simulink model "pro"  (R2012b)
settings: Solver=ode45  StartTime=0.0  StopTime=3  FixedStep=0.001  RelTol=1e-1  AbsTol=1e-2
undefined symbols (not defined in the file or in its folder): v_max
libraries: simulink x2
settings Model: Creator=Milos  LastModifiedBy=Caka
settings SolverCC: MaxConsecutiveMinStep=5

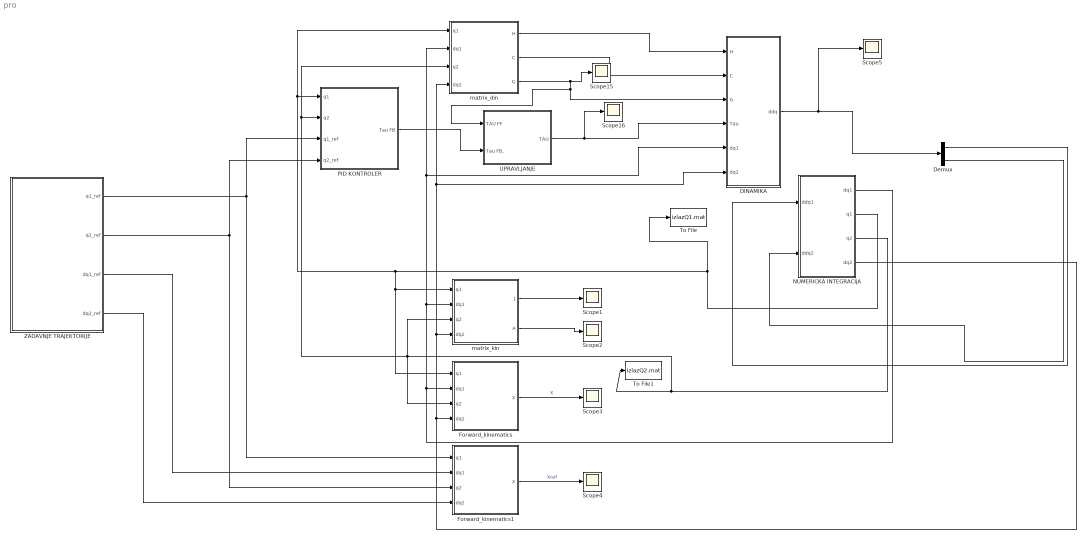
== system pro ==
  DINAMIKA : Subsystem
  Demux : Demux  Outputs=2
  Forward_kinematics : Subsystem
  Forward_kinematics1 : Subsystem
  NUMERICKA INTEGRACIjA : Subsystem
  PID KONTROLER : Subsystem
  Scope{1..5,15..16} (7 alike) : Scope
      Scope1 settings: TimeRange=5  YMin=0  YMax=70  SaveName=ScopeData4
      Scope15 settings: TimeRange=5  YMin=0  YMax=70  SaveName=ScopeData19
      Scope16 settings: TimeRange=5  YMin=0  YMax=70  SaveName=ScopeData20
      Scope2 settings: TimeRange=5  YMin=0  YMax=70  SaveName=ScopeData5
      Scope3 settings: TimeRange=5  YMin=0  YMax=70  SaveName=ScopeData6
      Scope4 settings: TimeRange=5  YMin=0  YMax=70  SaveName=ScopeData7
      Scope5 settings: TimeRange=5  YMin=0  YMax=70  SaveName=ScopeData9
  To File : ToFile  Filename=izlazQ1.mat  MatrixName=q1  SampleTime=0.01
  To File1 : ToFile  Filename=izlazQ2.mat  MatrixName=q2  SampleTime=0.01
  UPRAVLJANJE : Subsystem
  ZADAVNJE TRAJEKTORIJE : Subsystem
  matrix_din : Subsystem
  matrix_kin : Subsystem
  wires:
  matrix_din/3(G) -> Scope15/1, DINAMIKA/3(G), UPRAVLJANJE/1(TAU FF)
  matrix_kin/1(J) -> Scope1/1
  matrix_kin/2(A) -> Scope2/1
  Forward_kinematics/1(X) -> Scope3/1  "X"
  Forward_kinematics1/1(X) -> Scope4/1  "Xref"
  ZADAVNJE TRAJEKTORIJE/1(q1_ref) -> PID KONTROLER/3(q1_ref), Forward_kinematics1/1(q1)
  ZADAVNJE TRAJEKTORIJE/4(dq2_ref) -> Forward_kinematics1/4(dq2)
  matrix_din/1(H) -> DINAMIKA/1(H)
  matrix_din/2(C) -> DINAMIKA/2(C)
  UPRAVLJANJE/1(TAU) -> Scope16/1, DINAMIKA/4(Tau)
  PID KONTROLER/1("Tau FB ") -> UPRAVLJANJE/2(Tau FB,)
  ZADAVNJE TRAJEKTORIJE/2(q2_ref) -> PID KONTROLER/4(q2_ref), Forward_kinematics1/3(q2)
  ZADAVNJE TRAJEKTORIJE/3(dq1_ref) -> Forward_kinematics1/2(dq1)
  NUMERICKA INTEGRACIjA/4(dq2) -> Forward_kinematics/4(dq2), DINAMIKA/6(dq2), matrix_din/4(dq2), matrix_kin/4(dq2)
  NUMERICKA INTEGRACIjA/2(q1) -> Forward_kinematics/1(q1), matrix_kin/1(q1), matrix_din/1(q1), PID KONTROLER/1(q1), To File/1
  NUMERICKA INTEGRACIjA/3(q2) -> To File1/1, PID KONTROLER/2(q2), matrix_din/3(q2), matrix_kin/3(q2), Forward_kinematics/3(q2)
  Demux/1 -> NUMERICKA INTEGRACIjA/1(ddq1)
  Demux/2 -> NUMERICKA INTEGRACIjA/2(ddq2)
  NUMERICKA INTEGRACIjA/1(dq1) -> DINAMIKA/5(dq1), matrix_din/2(dq1), matrix_kin/2(dq1), Forward_kinematics/2(dq1)
  DINAMIKA/1(ddq) -> Scope5/1, Demux/1

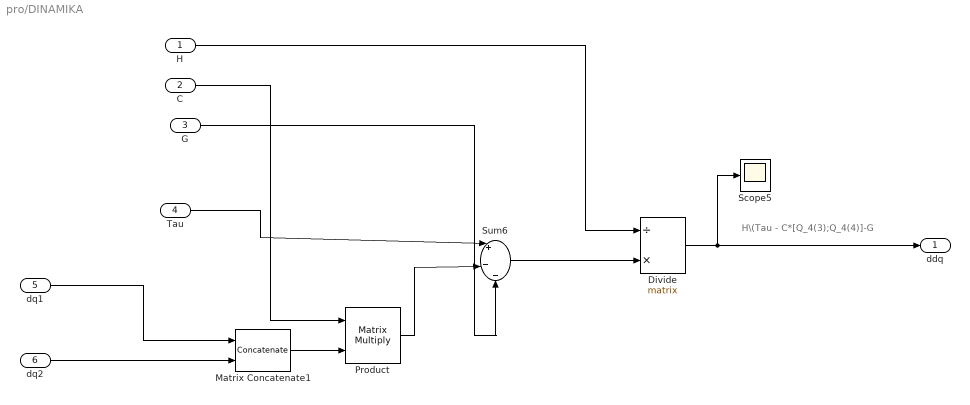
== system pro/DINAMIKA ==
  note: H\(Tau - C*[Q_4(3);Q_4(4)]-G
  H : Inport
  C : Inport  Port=2
  G : Inport  Port=3
  Tau : Inport  Port=4
  dq1 : Inport  Port=5
  dq2 : Inport  Port=6
  Divide : Product  Inputs=/*  Multiplication=Matrix(*)
  Matrix Concatenate1 : Concatenate  Mode=Multidimensional array
  Product : Product  Multiplication=Matrix(*)  RndMeth=Zero
  Scope5 : Scope
      settings: TimeRange=5  YMin=0  YMax=70  SaveName=ScopeData8
  Sum6 : Sum  Inputs=|+|-|-
  ddq : Outport
  wires:
  Product/1 -> Sum6/2
  H/1 -> Divide/1
  Matrix Concatenate1/1 -> Product/2
  Sum6/1 -> Divide/2
  C/1 -> Product/1
  Divide/1 -> ddq/1, Scope5/1
  Tau/1 -> Sum6/1
  G/1 -> Sum6/3
  dq1/1 -> Matrix Concatenate1/1
  dq2/1 -> Matrix Concatenate1/2

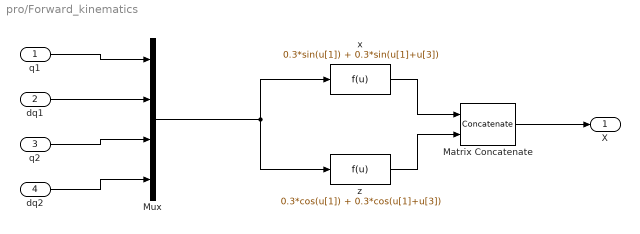
== system pro/Forward_kinematics ==
  q1 : Inport
  dq1 : Inport  Port=2
  q2 : Inport  Port=3
  dq2 : Inport  Port=4
  Matrix Concatenate : Concatenate  Mode=Multidimensional array
  Mux : Mux
  x : Fcn  Expr=0.3*sin(u[1]) + 0.3*sin(u[1]+u[3])
  z : Fcn  Expr=0.3*cos(u[1]) + 0.3*cos(u[1]+u[3])
  X : Outport
  wires:
  x/1 -> Matrix Concatenate/1
  z/1 -> Matrix Concatenate/2
  Matrix Concatenate/1 -> X/1
  q1/1 -> Mux/1
  dq1/1 -> Mux/2
  q2/1 -> Mux/3
  dq2/1 -> Mux/4
  Mux/1 -> x/1, z/1

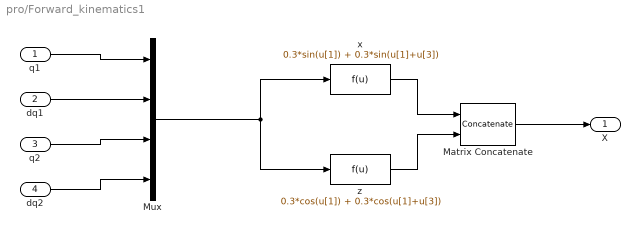
== system pro/Forward_kinematics1 ==
  q1 : Inport
  dq1 : Inport  Port=2
  q2 : Inport  Port=3
  dq2 : Inport  Port=4
  Matrix Concatenate : Concatenate  Mode=Multidimensional array
  Mux : Mux
  x : Fcn  Expr=0.3*sin(u[1]) + 0.3*sin(u[1]+u[3])
  z : Fcn  Expr=0.3*cos(u[1]) + 0.3*cos(u[1]+u[3])
  X : Outport
  wires:
  Mux/1 -> z/1, x/1
  dq2/1 -> Mux/4
  q2/1 -> Mux/3
  dq1/1 -> Mux/2
  q1/1 -> Mux/1
  Matrix Concatenate/1 -> X/1
  z/1 -> Matrix Concatenate/2
  x/1 -> Matrix Concatenate/1

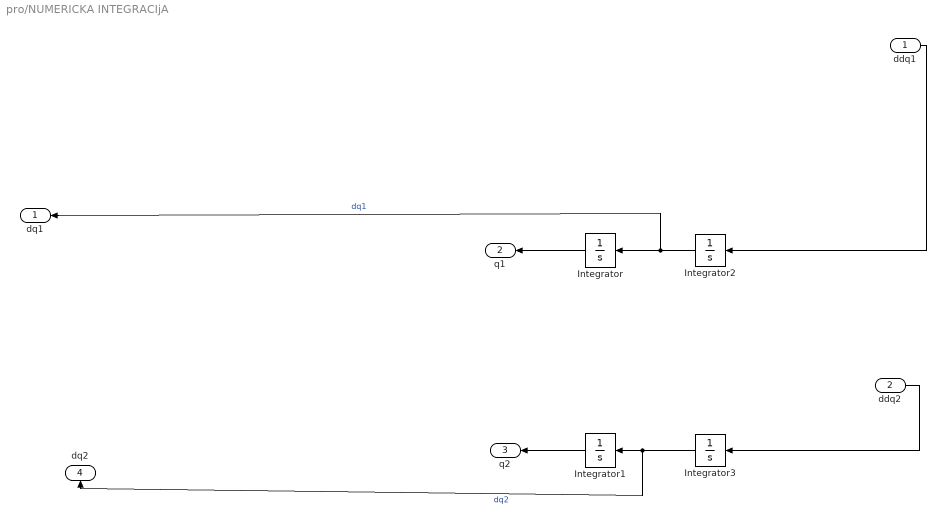
== system pro/NUMERICKA INTEGRACIjA ==
  ddq1 : Inport
  ddq2 : Inport  Port=2
  Integrator : Integrator  InitialCondition=30*pi/180  UpperSaturationLimit=3  LowerSaturationLimit=0  AbsoluteTolerance=1e-2
  Integrator1 : Integrator  InitialCondition=60*pi/180  UpperSaturationLimit=3  LowerSaturationLimit=0  AbsoluteTolerance=1e-2
  Integrator2 : Integrator  UpperSaturationLimit=3  LowerSaturationLimit=0  AbsoluteTolerance=1e-2
  Integrator3 : Integrator  UpperSaturationLimit=3  LowerSaturationLimit=0  AbsoluteTolerance=1e-2
  dq1 : Outport
  q1 : Outport  Port=2
  q2 : Outport  Port=3
  dq2 : Outport  Port=4
  wires:
  Integrator2/1 -> dq1/1, Integrator/1  "dq1"
  Integrator/1 -> q1/1
  Integrator3/1 -> dq2/1, Integrator1/1  "dq2"
  ddq1/1 -> Integrator2/1
  Integrator1/1 -> q2/1
  ddq2/1 -> Integrator3/1

== system pro/PID KONTROLER ==
  q1 : Inport
  q2 : Inport  Port=2
  q1_ref : Inport  Port=3
  q2_ref : Inport  Port=4
  Matrix Concatenate2 : Concatenate  Mode=Multidimensional array
  PID Controller (2DOF) : simulink/Continuous/PID Controller (2DOF)  Controller=PD  TimeDomain=Continuous-time  SampleTime=1  IntegratorMethod=Forward Euler  FilterMethod=Forward Euler  Form=Parallel  P=17  I=10  D=11  N=100  b=1  c=1  InitialConditionSource=internal  InitialConditionForIntegrator=0  InitialConditionForFilter=0  ExternalReset=none  LimitOutput=off  UpperSaturationLimit=inf  LowerSaturationLimit=-inf  LinearizeAsGain=on  AntiWindupMode=none  Kb=1  TrackingMode=off  Kt=1  PParamMin=[]  PParamMax=[]  IParamMin=[]  IParamMax=[]  DParamMin=[]  DParamMax=[]  NParamMin=[]  NParamMax=[]  bParamMin=[]  bParamMax=[]  cParamMin=[]  cParamMax=[]  KbParamMin=[]  KbParamMax=[]  KtParamMin=[]  KtParamMax=[]  POutMin=[]  POutMax=[]  IOutMin=[]  IOutMax=[]  DOutMin=[]  DOutMax=[]  NOutMin=[]  NOutMax=[]  bOutMin=[]  bOutMax=[]  cOutMin=[]  cOutMax=[]  KbOutMin=[]  KbOutMax=[]  KtOutMin=[]  KtOutMax=[]  IntegratorOutMin=[]  IntegratorOutMax=[]  FilterOutMin=[]  FilterOutMax=[]  SumOutMin=[]  SumOutMax=[]  Sum1OutMin=[]  Sum1OutMax=[]  Sum2OutMin=[]  Sum2OutMax=[]  Sum3OutMin=[]  Sum3OutMax=[]  SumI1OutMin=[]  SumI1OutMax=[]  SumI2OutMin=[]  SumI2OutMax=[]  SumI3OutMin=[]  SumI3OutMax=[]  SumDOutMin=[]  SumDOutMax=[]  SaturationOutMin=[]  SaturationOutMax=[]  IntegratorContinuousStateAttributes=''  IntegratorStateMustResolveToSignalObject=off  IntegratorRTWStateStorageClass=Auto  FilterContinuousStateAttributes=''  FilterStateMustResolveToSignalObject=off  FilterRTWStateStorageClass=Auto
  PID Controller (2DOF)1 : simulink/Continuous/PID Controller (2DOF)  Controller=PD  TimeDomain=Continuous-time  SampleTime=1  IntegratorMethod=Forward Euler  FilterMethod=Forward Euler  Form=Parallel  P=17  I=10  D=11  N=100  b=1  c=1  InitialConditionSource=internal  InitialConditionForIntegrator=0  InitialConditionForFilter=0  ExternalReset=none  LimitOutput=off  UpperSaturationLimit=inf  LowerSaturationLimit=-inf  LinearizeAsGain=on  AntiWindupMode=none  Kb=1  TrackingMode=off  Kt=1  PParamMin=[]  PParamMax=[]  IParamMin=[]  IParamMax=[]  DParamMin=[]  DParamMax=[]  NParamMin=[]  NParamMax=[]  bParamMin=[]  bParamMax=[]  cParamMin=[]  cParamMax=[]  KbParamMin=[]  KbParamMax=[]  KtParamMin=[]  KtParamMax=[]  POutMin=[]  POutMax=[]  IOutMin=[]  IOutMax=[]  DOutMin=[]  DOutMax=[]  NOutMin=[]  NOutMax=[]  bOutMin=[]  bOutMax=[]  cOutMin=[]  cOutMax=[]  KbOutMin=[]  KbOutMax=[]  KtOutMin=[]  KtOutMax=[]  IntegratorOutMin=[]  IntegratorOutMax=[]  FilterOutMin=[]  FilterOutMax=[]  SumOutMin=[]  SumOutMax=[]  Sum1OutMin=[]  Sum1OutMax=[]  Sum2OutMin=[]  Sum2OutMax=[]  Sum3OutMin=[]  Sum3OutMax=[]  SumI1OutMin=[]  SumI1OutMax=[]  SumI2OutMin=[]  SumI2OutMax=[]  SumI3OutMin=[]  SumI3OutMax=[]  SumDOutMin=[]  SumDOutMax=[]  SaturationOutMin=[]  SaturationOutMax=[]  IntegratorContinuousStateAttributes=''  IntegratorStateMustResolveToSignalObject=off  IntegratorRTWStateStorageClass=Auto  FilterContinuousStateAttributes=''  FilterStateMustResolveToSignalObject=off  FilterRTWStateStorageClass=Auto
  "Tau FB " : Outport
  wires:
  PID Controller (2DOF)1/1 -> Matrix Concatenate2/2
  PID Controller (2DOF)/1 -> Matrix Concatenate2/1
  q1/1 -> PID Controller (2DOF)/2
  q1_ref/1 -> PID Controller (2DOF)/1
  q2/1 -> PID Controller (2DOF)1/2
  q2_ref/1 -> PID Controller (2DOF)1/1
  Matrix Concatenate2/1 -> "Tau FB "/1

== system pro/UPRAVLJANJE ==
  note: TAU FF
  TAU FF : Inport
  Tau FB, : Inport  Port=2
  Sum3 : Sum  Inputs=|++
  TAU : Outport
  wires:
  Tau FB,/1 -> Sum3/2
  Sum3/1 -> TAU/1  "TAU"
  TAU FF/1 -> Sum3/1

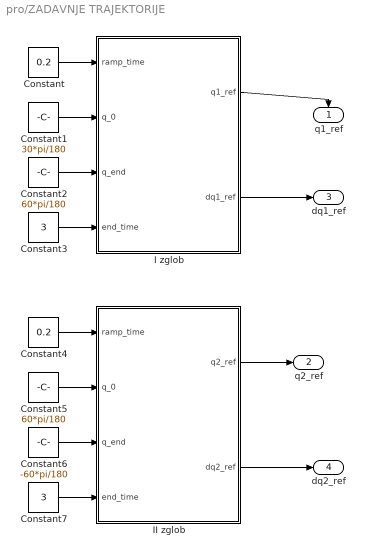
== system pro/ZADAVNJE TRAJEKTORIJE ==
  Constant : Constant  Value=0.2
  Constant1 : Constant  Value=30*pi/180
  Constant2 : Constant  Value=60*pi/180
  Constant3 : Constant  Value=3
  Constant4 : Constant  Value=0.2
  Constant5 : Constant  Value=60*pi/180
  Constant6 : Constant  Value=-60*pi/180
  Constant7 : Constant  Value=3
  I zglob : Subsystem
  II zglob : Subsystem
  q1_ref : Outport
  q2_ref : Outport  Port=2
  dq1_ref : Outport  Port=3
  dq2_ref : Outport  Port=4
  wires:
  Constant/1 -> I zglob/1(ramp_time)
  Constant3/1 -> I zglob/4(end_time)
  Constant2/1 -> I zglob/3(q_end)
  Constant4/1 -> II zglob/1(ramp_time)
  Constant7/1 -> II zglob/4(end_time)
  Constant6/1 -> II zglob/3(q_end)
  Constant5/1 -> II zglob/2(q_0)
  Constant1/1 -> I zglob/2(q_0)
  II zglob/1(q2_ref) -> q2_ref/1
  I zglob/1(q1_ref) -> q1_ref/1
  II zglob/2(dq2_ref) -> dq2_ref/1
  I zglob/2(dq1_ref) -> dq1_ref/1

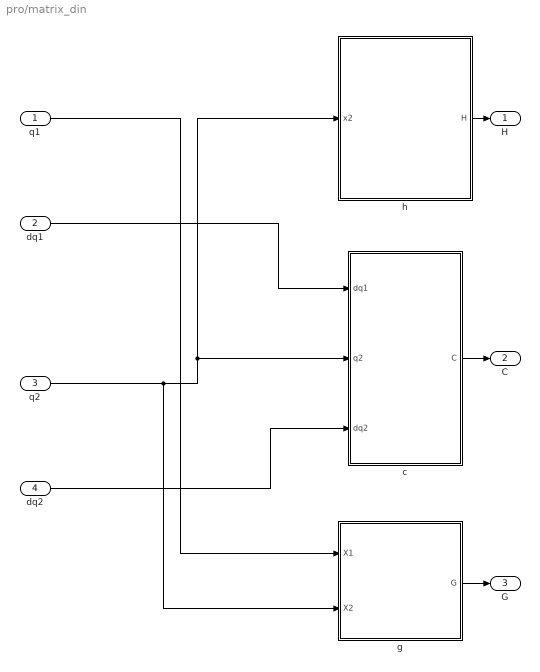
== system pro/matrix_din ==
  q1 : Inport
  dq1 : Inport  Port=2
  q2 : Inport  Port=3
  dq2 : Inport  Port=4
  c : Subsystem
  g : Subsystem
  h : Subsystem
  H : Outport
  C : Outport  Port=2
  G : Outport  Port=3
  wires:
  h/1(H) -> H/1
  q2/1 -> g/2(X2), h/1(x2), c/2(q2)
  q1/1 -> g/1(X1)
  dq1/1 -> c/1(dq1)
  dq2/1 -> c/3(dq2)
  g/1(G) -> G/1
  c/1(C) -> C/1

== system pro/matrix_kin ==
  q1 : Inport
  dq1 : Inport  Port=2
  q2 : Inport  Port=3
  dq2 : Inport  Port=4
  a : Subsystem
  jot : Subsystem
  J : Outport
  A : Outport  Port=2
  wires:
  jot/1(J) -> J/1
  q1/1 -> jot/1(x1), a/1(X1)
  q2/1 -> a/3(X2), jot/2(x2)
  dq2/1 -> a/4(dX2)
  a/1(A) -> A/1
  dq1/1 -> a/2(dX1)

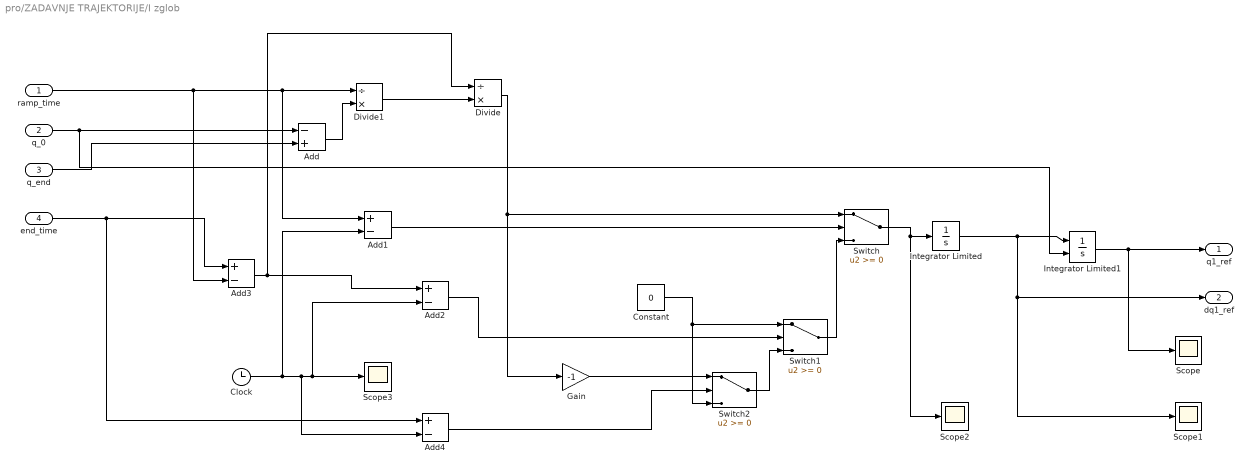
== system pro/ZADAVNJE TRAJEKTORIJE/I zglob ==
  ramp_time : Inport
  q_0 : Inport  Port=2
  q_end : Inport  Port=3
  end_time : Inport  Port=4
  Add : Sum  Inputs=-+
  Add{1..4} (4 alike) : Sum  Inputs=+-
  Clock : Clock
  Constant : Constant  Value=0
  Divide : Product  Inputs=/*
  Divide1 : Product  Inputs=/*
  Gain : Gain  Gain=-1
  Integrator Limited : Integrator  UpperSaturationLimit=v_max  LowerSaturationLimit=-v_max
  Integrator Limited1 : Integrator  InitialConditionSource=external  UpperSaturationLimit=v_max  LowerSaturationLimit=-v_max
  Scope{,1..3} (4 alike) : Scope
      Scope settings: TimeRange=1  YMin=0  YMax=200
      Scope2 settings: YMin=-20  SaveName=ScopeData2
      Scope3 settings: YMax=15  SaveName=ScopeData3
  Switch : Switch
  Switch1 : Switch
  Switch2 : Switch
  q1_ref : Outport
  dq1_ref : Outport  Port=2
  wires:
  Divide/1 -> Gain/1, Switch/1
  q_end/1 -> Add/2
  Divide1/1 -> Divide/2
  Add/1 -> Divide1/2
  Switch/1 -> Scope2/1, Integrator Limited/1
  Add1/1 -> Switch/2
  ramp_time/1 -> Add3/2, Add1/1, Divide1/1
  Clock/1 -> Add4/2, Add2/2, Scope3/1, Add1/2
  Integrator Limited/1 -> dq1_ref/1, Scope1/1, Integrator Limited1/1
  Integrator Limited1/1 -> q1_ref/1, Scope/1
  Switch1/1 -> Switch/3
  end_time/1 -> Add4/1, Add3/1
  Add3/1 -> Divide/1, Add2/1
  Add2/1 -> Switch1/2
  Constant/1 -> Switch2/3, Switch1/1
  Switch2/1 -> Switch1/3
  Add4/1 -> Switch2/2
  Gain/1 -> Switch2/1
  q_0/1 -> Integrator Limited1/2, Add/1

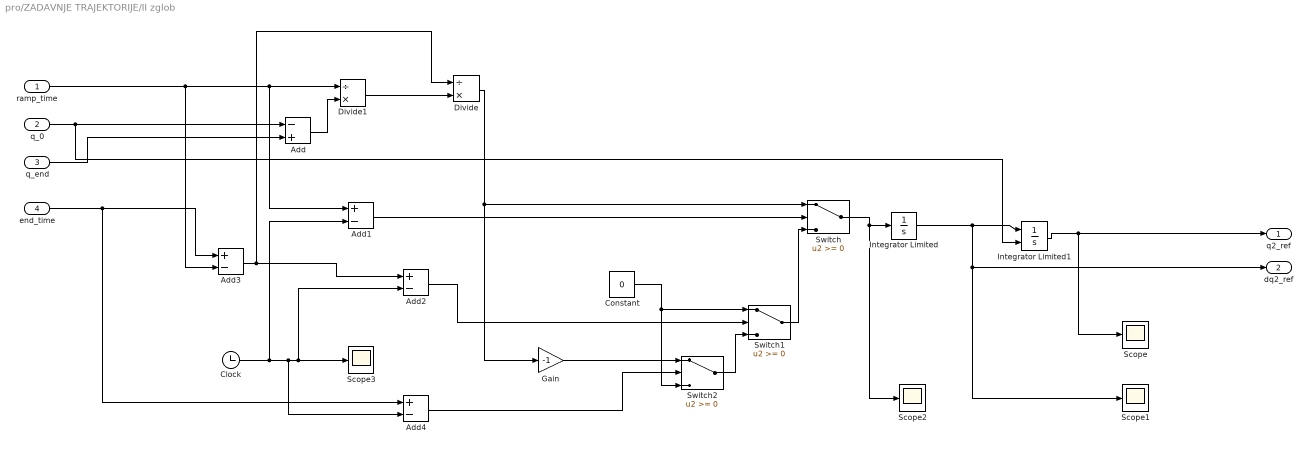
== system pro/ZADAVNJE TRAJEKTORIJE/II zglob ==
  ramp_time : Inport
  q_0 : Inport  Port=2
  q_end : Inport  Port=3
  end_time : Inport  Port=4
  Add : Sum  Inputs=-+
  Add{1..4} (4 alike) : Sum  Inputs=+-
  Clock : Clock
  Constant : Constant  Value=0
  Divide : Product  Inputs=/*
  Divide1 : Product  Inputs=/*
  Gain : Gain  Gain=-1
  Integrator Limited : Integrator  UpperSaturationLimit=v_max  LowerSaturationLimit=-v_max
  Integrator Limited1 : Integrator  InitialConditionSource=external  UpperSaturationLimit=v_max  LowerSaturationLimit=-v_max
  Scope{,1..3} (4 alike) : Scope
      Scope settings: TimeRange=1  YMin=0  YMax=200
      Scope2 settings: YMin=-20  SaveName=ScopeData2
      Scope3 settings: YMax=15  SaveName=ScopeData3
  Switch : Switch
  Switch1 : Switch
  Switch2 : Switch
  q2_ref : Outport
  dq2_ref : Outport  Port=2
  wires:
  Divide/1 -> Gain/1, Switch/1
  q_end/1 -> Add/2
  Divide1/1 -> Divide/2
  Add/1 -> Divide1/2
  Switch/1 -> Scope2/1, Integrator Limited/1
  Add1/1 -> Switch/2
  ramp_time/1 -> Add3/2, Add1/1, Divide1/1
  Clock/1 -> Add4/2, Add2/2, Scope3/1, Add1/2
  Integrator Limited/1 -> dq2_ref/1, Scope1/1, Integrator Limited1/1
  Integrator Limited1/1 -> q2_ref/1, Scope/1
  Switch1/1 -> Switch/3
  end_time/1 -> Add4/1, Add3/1
  Add3/1 -> Divide/1, Add2/1
  Add2/1 -> Switch1/2
  Constant/1 -> Switch2/3, Switch1/1
  Switch2/1 -> Switch1/3
  Add4/1 -> Switch2/2
  Gain/1 -> Switch2/1
  q_0/1 -> Integrator Limited1/2, Add/1

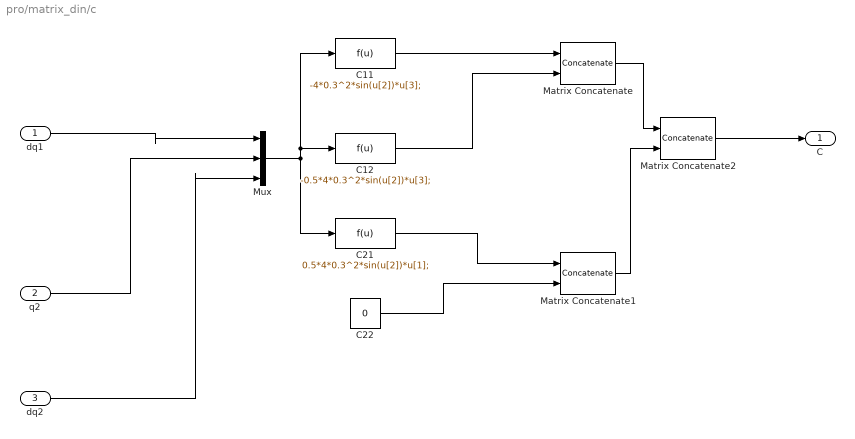
== system pro/matrix_din/c ==
  dq1 : Inport
  q2 : Inport  Port=2
  dq2 : Inport  Port=3
  C11 : Fcn  Expr=-4*0.3^2*sin(u[2])*u[3];
  C12 : Fcn  Expr=-0.5*4*0.3^2*sin(u[2])*u[3];
  C21 : Fcn  Expr=0.5*4*0.3^2*sin(u[2])*u[1];
  C22 : Constant  Value=0
  Matrix Concatenate : Concatenate  Mode=Multidimensional array  ConcatenateDimension=2
  Matrix Concatenate1 : Concatenate  Mode=Multidimensional array  ConcatenateDimension=2
  Matrix Concatenate2 : Concatenate  Mode=Multidimensional array
  Mux : Mux  Inputs=3
  C : Outport
  wires:
  q2/1 -> Mux/2
  dq1/1 -> Mux/1
  Mux/1 -> C11/1, C12/1, C21/1
  dq2/1 -> Mux/3
  C21/1 -> Matrix Concatenate1/1
  Matrix Concatenate/1 -> Matrix Concatenate2/1
  C12/1 -> Matrix Concatenate/2
  Matrix Concatenate1/1 -> Matrix Concatenate2/2
  C22/1 -> Matrix Concatenate1/2
  C11/1 -> Matrix Concatenate/1
  Matrix Concatenate2/1 -> C/1

== system pro/matrix_din/g ==
  X1 : Inport
  X2 : Inport  Port=2
  G11 : Fcn  Expr=-1.5*4*0.3*9.81*sin(u[1])-0.5*4*0.3*9.81*sin(u[1]+u[2])
  G21 : Fcn  Expr=-0.5*4*0.3*9.81*sin(u[1]+u[2])
  Matrix Concatenate : Concatenate  Mode=Multidimensional array
  Mux : Mux  Inputs=2
  G : Outport
  wires:
  G11/1 -> Matrix Concatenate/1
  G21/1 -> Matrix Concatenate/2
  X1/1 -> Mux/1
  Matrix Concatenate/1 -> G/1
  Mux/1 -> G21/1, G11/1
  X2/1 -> Mux/2

== system pro/matrix_din/h ==
  x2 : Inport
  Constant8 : Constant  Value=0.03+0.25*4*0.3^2
  H11 : Fcn  Expr=2*0.03+4*0.3^2*(1.5+cos(u[1]))
  H12 : Fcn  Expr=0.03+0.5*4*0.3^2*(0.5+cos(u[1]))
  Matrix Concatenate : Concatenate  Mode=Multidimensional array  ConcatenateDimension=2
  Matrix Concatenate1 : Concatenate  Mode=Multidimensional array  ConcatenateDimension=2
  Matrix Concatenate2 : Concatenate  Mode=Multidimensional array
  H : Outport
  wires:
  Matrix Concatenate2/1 -> H/1
  Matrix Concatenate/1 -> Matrix Concatenate2/1
  Matrix Concatenate1/1 -> Matrix Concatenate2/2
  Constant8/1 -> Matrix Concatenate1/2
  H12/1 -> Matrix Concatenate/2, Matrix Concatenate1/1
  x2/1 -> H12/1, H11/1
  H11/1 -> Matrix Concatenate/1

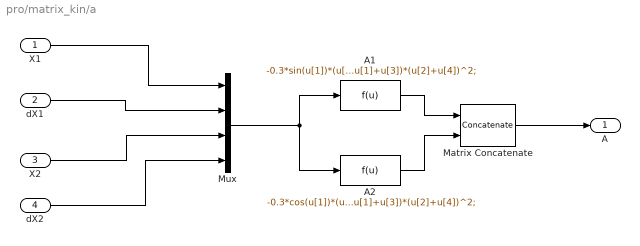
== system pro/matrix_kin/a ==
  X1 : Inport
  dX1 : Inport  Port=2
  X2 : Inport  Port=3
  dX2 : Inport  Port=4
  A1 : Fcn  Expr=-0.3*sin(u[1])*(u[2]^2)-0.3*sin(u[1]+u[3])*(u[2]+u[4])^2;
  A2 : Fcn  Expr=-0.3*cos(u[1])*(u[2]^2)-0.3*cos(u[1]+u[3])*(u[2]+u[4])^2;
  Matrix Concatenate : Concatenate  Mode=Multidimensional array
  Mux : Mux
  A : Outport
  wires:
  A2/1 -> Matrix Concatenate/2
  Matrix Concatenate/1 -> A/1
  X2/1 -> Mux/3
  X1/1 -> Mux/1
  Mux/1 -> A2/1, A1/1
  A1/1 -> Matrix Concatenate/1
  dX1/1 -> Mux/2
  dX2/1 -> Mux/4

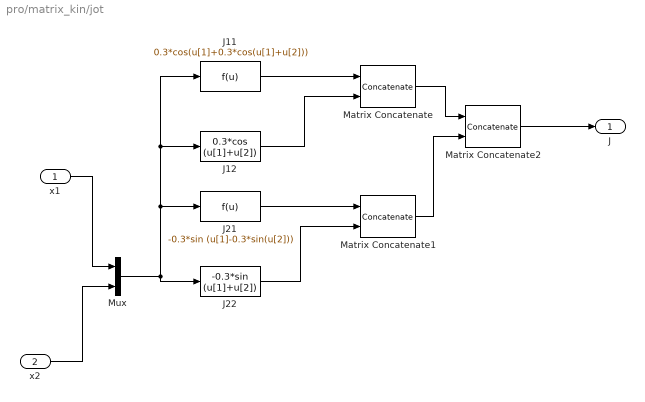
== system pro/matrix_kin/jot ==
  x1 : Inport
  x2 : Inport  Port=2
  J11 : Fcn  Expr=0.3*cos(u[1]+0.3*cos(u[1]+u[2]))
  J12 : Fcn  Expr=0.3*cos (u[1]+u[2])
  J21 : Fcn  Expr=-0.3*sin (u[1]-0.3*sin(u[2]))
  J22 : Fcn  Expr=-0.3*sin (u[1]+u[2])
  Matrix Concatenate : Concatenate  Mode=Multidimensional array  ConcatenateDimension=2
  Matrix Concatenate1 : Concatenate  Mode=Multidimensional array  ConcatenateDimension=2
  Matrix Concatenate2 : Concatenate  Mode=Multidimensional array
  Mux : Mux  Inputs=2
  J : Outport
  wires:
  J11/1 -> Matrix Concatenate/1
  Mux/1 -> J21/1, J11/1, J12/1, J22/1
  Matrix Concatenate1/1 -> Matrix Concatenate2/2
  J21/1 -> Matrix Concatenate1/1
  J22/1 -> Matrix Concatenate1/2
  Matrix Concatenate/1 -> Matrix Concatenate2/1
  x1/1 -> Mux/1
  Matrix Concatenate2/1 -> J/1
  J12/1 -> Matrix Concatenate/2
  x2/1 -> Mux/2
